simulink model "cstr_nmpc_ctrl"  (R2020a)
settings: Solver=ode45  StartTime=0  StopTime=200  MaxStep=0.5*Ts  RelTol=1e-3  EnableMultiTasking=on
values from neighbouring files (symbols this model uses):
  Ts = 0.1    [stateFcn.m]
undefined symbols (not defined in the file or in its folder): CA0, ny, R, u0, x0
libraries: mympclib x2, simulink x1
settings Model: Creator=The MathWorks, Inc.  LastModifiedBy=kohei
settings DataIOCC: ExternalInput=ExtIn  InitialState=[311.267; 8.5695]  SaveFormat=Structure  SaveOutput=off  SaveTime=off  ReturnWorkspaceOutputs=off  SignalLoggingName=logsOut
settings OptimizationCC: BooleanDataType=off  DefaultParameterBehavior=Inlined  InlineInvariantSignals=on  BufferReuse=off  ExpressionDepthLimit=2147483647  InitFltsAndDblsToZero=on  LifeSpan=inf
settings DebuggingCC: SaveWithParameterizedLinksMsg=none  UnderspecifiedInitializationDetection=Classic  MergeDetectMultiDrivingBlocksExec=none  CheckExecutionContextPreStartOutputMsg=on  CheckExecutionContextRuntimeOutputMsg=on  SignalResolutionControl=TryResolveAllWithWarning  MultiTaskDSMMsg=warning  MultiTaskCondExecSysMsg=none  StateNameClashWarn=warning  SFUnexpectedBacktrackingDiag=warning  SFNoUnconditionalDefaultTransitionDiag=warning  SFExecutionAtInitializationDiag=none  ArithmeticOperatorsInVariantConditions=warning
settings HardwareCC: ProdBitPerPointer=32  ProdBitPerSizeT=32  ProdBitPerPtrDiffT=32  ProdLargestAtomicFloat=None  ProdIntDivRoundTo=Undefined  ProdEndianess=Unspecified  ProdWordSize=32  ProdHWDeviceType=32-bit Generic  TargetBitPerPointer=64  TargetBitPerSizeT=64  TargetBitPerPtrDiffT=64  TargetLongLongMode=on  TargetIntDivRoundTo=Zero  TargetEndianess=LittleEndian  TargetWordSize=64  TargetHWDeviceType=MATLAB Host  ProdEqTarget=off
settings ModelReferenceCC: PropagateSignalLabelsOutOfModel=off
settings SFSimCC: SimUseLocalCustomCode=off  CustomCodeUndefinedFunction=UseInterfaceOnly
settings RTWCC: RTWUseLocalCustomCode=off
settings CodeAppCC: StateflowObjectComments=on
settings GRTTargetCC: TargetFcnLib=ansi_tfl_tmw.mat  TargetLangStandard=C89/C90 (ANSI)  CombineOutputUpdateFcns=off  GRTInterface=on
settings ConfigComp: CovMetricSettings=dw  CovHtmlReporting=on  CovSaveCumulativeToWorkspaceVar=on  CovSaveSingleToWorkspaceVar=on  CovExternalEMLEnable=off  CovSFcnEnable=off

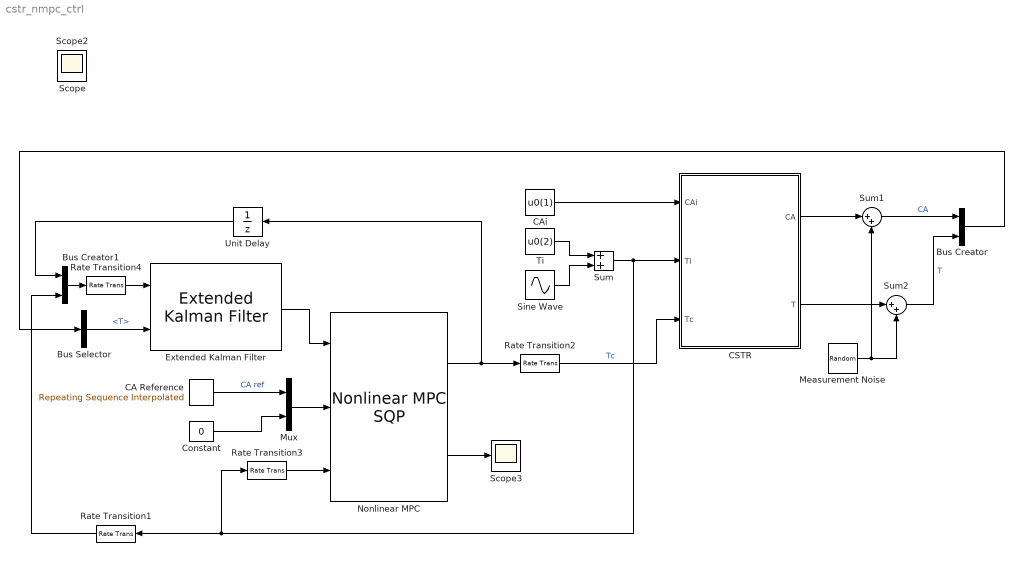
== system cstr_nmpc_ctrl ==
  Bus Creator : BusCreator  Inputs=2
  Bus Creator1 : BusCreator  Inputs=2
  Bus Selector : BusSelector  OutputSignals=T
  CA Reference : simulink/Sources/Repeating Sequence Interpolated  OutValues=[CA0,CA0, 2, 2]  TimeValues="[0 50  150 200]"  LookUpMeth=Interpolation-Use End Values  tsamp=Ts  OutMin=[]  OutMax=[]  OutDataTypeStr=double  OutputDataTypeScalingMode=double  OutDataType=fixdt(0,8)  OutScaling=2^-10
  CAi : Constant  Value=u0(1)
  CSTR : Subsystem
  Constant : Constant  Value=0
  Extended Kalman Filter : mympclib/Extended Kalman Filter  stateFunction='f'  jacobianStateFunction='A'  measurementFunction='h'  jacobianMeasurmentFunction='C'  Bv=Bv  Q=Q  R=R  xhat0=xhat0  P0=P0  Ts=Ts  numState=nx  numOutput=ny-1  enableP=off  enableG=off
      settings: SourceProductName=My MPC Library
  Measurement Noise : RandomNumber  Variance=0.001  SampleTime=Ts
  Mux : Mux  Inputs=2
  Nonlinear MPC : mympclib/Nonlinear MPC SQP  params=params  ny=ny  nu=nu  Ts=Ts  enableDist=on  nd=nd  enableSlack=off  enableStatus=on
      settings: SourceProductName=My MPC Library
  Rate Transition1 : RateTransition  InitialCondition=u0(2)
  Rate Transition2 : RateTransition  InitialCondition=u0(3)
  Rate Transition3 : RateTransition  InitialCondition=u0(2)
  Rate Transition4 : RateTransition  InitialCondition=[u0(3);u0(2)]
  Scope3 : Scope
  Sine Wave : Sin  Frequency=0.1  SampleTime=0
  Sum : Sum
  Sum1 : Sum  Inputs=|++
  Sum2 : Sum  Inputs=|++
  Ti : Constant  Value=u0(2)
  Unit Delay : UnitDelay  InitialCondition=u0(3)  SampleTime=-1  HasFrameUpgradeWarning=on
  Scope : Scope
  Scope2 : Scope
  wires:
  CAi/1 -> CSTR/1(CAi)
  Ti/1 -> Sum/1
  Sine Wave/1 -> Sum/2
  CSTR/2(T) -> Sum2/1
  CSTR/1(CA) -> Sum1/1
  Measurement Noise/1 -> Sum2/2, Sum1/2
  Nonlinear MPC/1 -> Unit Delay/1, Rate Transition2/1
  Sum/1 -> CSTR/2(Ti), Rate Transition1/1, Rate Transition3/1
  Rate Transition2/1 -> CSTR/3(Tc)  "Tc"
  CA Reference/1 -> Mux/1  "CA ref"
  Constant/1 -> Mux/2
  Sum1/1 -> Bus Creator/1  "CA"
  Sum2/1 -> Bus Creator/2  "T"
  Extended Kalman Filter/1 -> Nonlinear MPC/1
  Mux/1 -> Nonlinear MPC/2
  Rate Transition3/1 -> Nonlinear MPC/3
  Nonlinear MPC/2 -> Scope3/1
  Bus Selector/1 -> Extended Kalman Filter/2  "<T>"
  Bus Creator/1 -> Bus Selector/1
  Bus Creator1/1 -> Rate Transition4/1
  Rate Transition4/1 -> Extended Kalman Filter/1
  Unit Delay/1 -> Bus Creator1/1
  Rate Transition1/1 -> Bus Creator1/2

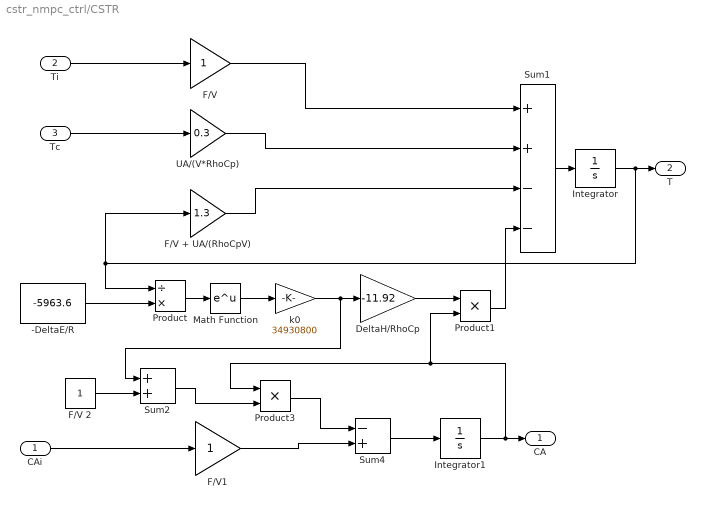
== system cstr_nmpc_ctrl/CSTR ==
  CAi : Inport
  Ti : Inport  Port=2
  Tc : Inport  Port=3
  -DeltaE/R : Constant  Value=-5963.6
  DeltaH/RhoCp : Gain  Gain=-11.92  SaturateOnIntegerOverflow=on  OutDataTypeStr=Inherit: Same as input  ParamDataTypeStr=Inherit: Same as input
  F/V : Gain  SaturateOnIntegerOverflow=on  OutDataTypeStr=Inherit: Same as input  ParamDataTypeStr=Inherit: Same as input
  F/V + UA/(RhoCpV) : Gain  Gain=1.3  SaturateOnIntegerOverflow=on  OutDataTypeStr=Inherit: Same as input  ParamDataTypeStr=Inherit: Same as input
  F/V 2 : Constant
  F/V1 : Gain  SaturateOnIntegerOverflow=on  OutDataTypeStr=Inherit: Same as input  ParamDataTypeStr=Inherit: Same as input
  Integrator : Integrator  InitialCondition=x0(2)  LimitOutput=on  LowerSaturationLimit=0
  Integrator1 : Integrator  InitialCondition=x0(1)  LimitOutput=on  LowerSaturationLimit=0
  Math Function : Math  SignedPower=on  SaturateOnIntegerOverflow=on
  Product : Product  Inputs=/*  InputSameDT=on  RndMeth=Zero  SaturateOnIntegerOverflow=on  OutDataTypeStr=Inherit: Same as first input
  Product1 : Product  InputSameDT=on  RndMeth=Zero  SaturateOnIntegerOverflow=on  OutDataTypeStr=Inherit: Same as first input
  Product3 : Product  InputSameDT=on  RndMeth=Zero  SaturateOnIntegerOverflow=on  OutDataTypeStr=Inherit: Same as first input
  Sum1 : Sum  Inputs=++--  InputSameDT=on  SaturateOnIntegerOverflow=on  OutDataTypeStr=Inherit: Same as first input
  Sum2 : Sum  InputSameDT=on  SaturateOnIntegerOverflow=on  OutDataTypeStr=Inherit: Same as first input
  Sum4 : Sum  Inputs=-+  InputSameDT=on  SaturateOnIntegerOverflow=on  OutDataTypeStr=Inherit: Same as first input
  UA/(V*RhoCp) : Gain  Gain=0.3  SaturateOnIntegerOverflow=on  OutDataTypeStr=Inherit: Same as input  ParamDataTypeStr=Inherit: Same as input
  k0 : Gain  Gain=34930800  SaturateOnIntegerOverflow=on  OutDataTypeStr=Inherit: Same as input  ParamDataTypeStr=Inherit: Same as input
  CA : Outport
  T : Outport  Port=2
  wires:
  Sum2/1 -> Product3/2
  Tc/1 -> UA/(V*RhoCp)/1
  CAi/1 -> F/V1/1
  Ti/1 -> F/V/1
  F/V1/1 -> Sum4/2
  F/V 2/1 -> Sum2/2
  Integrator1/1 -> CA/1, Product3/1, Product1/2
  Sum4/1 -> Integrator1/1
  Product3/1 -> Sum4/1
  -DeltaE/R/1 -> Product/2
  k0/1 -> Sum2/1, DeltaH/RhoCp/1
  Product1/1 -> Sum1/4
  DeltaH/RhoCp/1 -> Product1/1
  Math Function/1 -> k0/1
  Product/1 -> Math Function/1
  F/V + UA/(RhoCpV)/1 -> Sum1/3
  UA/(V*RhoCp)/1 -> Sum1/2
  Integrator/1 -> T/1, F/V + UA/(RhoCpV)/1, Product/1
  Sum1/1 -> Integrator/1
  F/V/1 -> Sum1/1
